simulink model "sfcndemo_timestwo"  (Simulink 6.0)
settings: Solver=FixedStepDiscrete  StartTime=0.0  StopTime=10.0  RelTol=1e-3
settings Model: Creator=The MathWorks Inc.  LastModifiedBy=batserve  ExtModeTrigMode=oneshot  ExtModeArmWhenConnect=off  ExtModeAutoUpdateStatusClock=off
settings DataIOCC: LimitDataPoints=off
settings OptimizationCC: BooleanDataType=off
settings DebuggingCC: CheckExecutionContextPreStartOutputMsg=on  CheckExecutionContextRuntimeOutputMsg=on  SolverPrmCheckMsg=none
settings HardwareCC: TargetUnknown=on

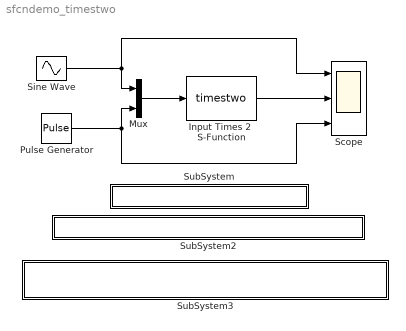
== system sfcndemo_timestwo ==
  Input Times 2  S-Function : S-Function  FunctionName=timestwo
      mask Type: S-function: timestwo
      mask Description: This is a C S-function which multiply input by two.
      mask Display:
      | plot([0 1 2 3 4 5 6 5 4 3 2 1 0 0],[0 .5 1 1.5 2 2.5 3 3.5 4 4.5 5 5.5 6 0]);
      | disp('2      ');
  Mux : Mux  Inputs=2
  Pulse Generator : DiscretePulseGenerator  PulseType=Time based  Amplitude=1:3  Period=1  PulseWidth=50
  Scope : Scope  NumInputPorts=3
      settings: TimeRange=10  YMin=-2~-5~0  YMax=2~10~3
  Sine Wave : Sin  Amplitude=1:2  SampleTime=0
  SubSystem : Subsystem  PropExecContextAcrossSSBoundary=on
      settings: OpenFcn=edit(fullfile(matlabroot,'simulink','src','timestwo.c'))
      mask Display: disp('matlabroot\simulink\src\timestwo.c');
  SubSystem2 : Subsystem  PropExecContextAcrossSSBoundary=on
      settings: OpenFcn=edit(fullfile(matlabroot,'toolbox','simulink','blocks','tlc_c','timestwo.tlc'))
      mask Display: disp('matlabroot\toolbox\simulink\blocks\tlc_c\timestwo.tlc');
  SubSystem3 : Subsystem  PropExecContextAcrossSSBoundary=on
      settings: OpenFcn=edit(fullfile(matlabroot,'toolbox','simulink','blocks','timestwo.m'))
      mask Display: disp('M-file: matlabroot\toolbox\simulink\blocks\timestwo.m\nNote:to run the m-file, please disable the executable mex file in your path.');
  wires:
  Input Times 2  S-Function/1 -> Scope/2
  Mux/1 -> Input Times 2  S-Function/1
  Pulse Generator/1 -> Mux/2, Scope/3
  Sine Wave/1 -> Mux/1, Scope/1

== system sfcndemo_timestwo/SubSystem ==

== system sfcndemo_timestwo/SubSystem2 ==

== system sfcndemo_timestwo/SubSystem3 ==
